simulink model "modeloNoLinealEcuaciones"  (Simulink 7.9)
settings: Solver=ode45  StartTime=0.0  StopTime=300  RelTol=1e-3
values from neighbouring files (symbols this model uses):
  K = lqr(A,B,Q,R)    [LQR.m]    (also in bestQ.m = setK_lqr(Q_i); graficosPenduloReal.m = setK_lqr(Q_optimo))
settings Model: Creator=gdiazh  LastModifiedBy=root
settings OptimizationCC: InitFltsAndDblsToZero=on
settings DebuggingCC: FcnCallInpInsideContextMsg=Use local settings  StrictBusMsg=Warning
settings SFSimCC: SimParseCustomCode=off
settings GRTTargetCC: CombineOutputUpdateFcns=off  GRTInterface=on

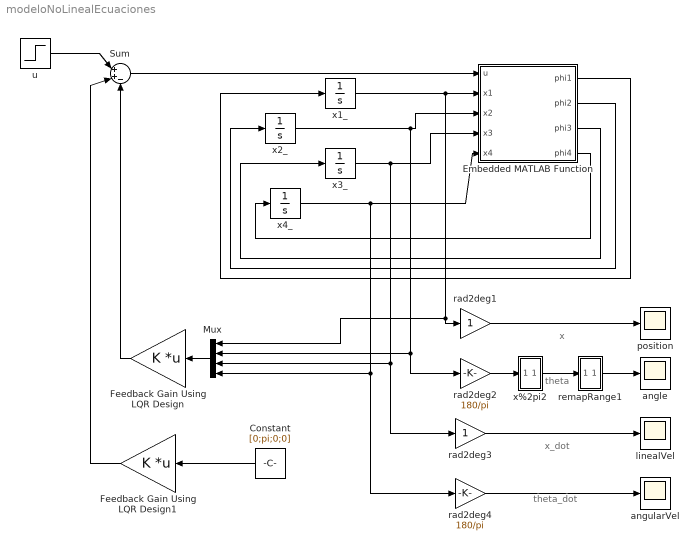
== system modeloNoLinealEcuaciones ==
  note: x
  note: theta
  note: x_dot
  note: theta_dot
  Constant : Constant  Value=[0;pi;0;0]  VectorParams1D=off
  Embedded MATLAB Function : MATLAB Function  TreatAsAtomicUnit=on
  Feedback Gain Using LQR Design : Gain  Gain=K  Multiplication=Matrix(K*u) (u vector)
  Feedback Gain Using LQR Design1 : Gain  Gain=K  Multiplication=Matrix(K*u) (u vector)
  Mux : Mux
  Sum : Sum  Inputs=|++-
  angle : Scope
      settings: TimeRange=0.35  YMin=89.75  YMax=90.25  SaveName=angle
  angularVel : Scope
      settings: SaveName=angularVel
  linealVel : Scope
      settings: SaveName=linealVel
  position : Scope
      settings: SaveName=position
  rad2deg1 : Gain  SaturateOnIntegerOverflow=on  OutDataTypeStr=Inherit: Same as input  ParamDataTypeStr=Inherit: Same as input
  rad2deg2 : Gain  Gain=180/pi  SaturateOnIntegerOverflow=on  OutDataTypeStr=Inherit: Same as input  ParamDataTypeStr=Inherit: Same as input
  rad2deg3 : Gain  SaturateOnIntegerOverflow=on  OutDataTypeStr=Inherit: Same as input  ParamDataTypeStr=Inherit: Same as input
  rad2deg4 : Gain  Gain=180/pi  SaturateOnIntegerOverflow=on  OutDataTypeStr=Inherit: Same as input  ParamDataTypeStr=Inherit: Same as input
  remapRange1 : MATLAB Function  TreatAsAtomicUnit=on
  u : Step  Time=0  After=4.7/1.88  SampleTime=0
  x%2pi2 : MATLAB Function  TreatAsAtomicUnit=on
  x1_ : Integrator  UpperSaturationLimit=50  LowerSaturationLimit=-50
  x2_ : Integrator  InitialCondition=200*pi/180  UpperSaturationLimit=2*pi  LowerSaturationLimit=0
  x3_ : Integrator  UpperSaturationLimit=100  LowerSaturationLimit=-100
  x4_ : Integrator  UpperSaturationLimit=100  LowerSaturationLimit=-100
  wires:
  Sum/1 -> Embedded MATLAB Function/1(u)
  Embedded MATLAB Function/1(phi1) -> x1_/1
  Embedded MATLAB Function/2(phi2) -> x2_/1
  Embedded MATLAB Function/3(phi3) -> x3_/1
  Embedded MATLAB Function/4(phi4) -> x4_/1
  rad2deg4/1 -> angularVel/1
  rad2deg3/1 -> linealVel/1
  rad2deg1/1 -> position/1
  remapRange1/1(y) -> angle/1
  x1_/1 -> Embedded MATLAB Function/2(x1), rad2deg1/1, Mux/1
  x2_/1 -> Embedded MATLAB Function/3(x2), rad2deg2/1, Mux/2
  x3_/1 -> Embedded MATLAB Function/4(x3), rad2deg3/1, Mux/3
  x4_/1 -> Embedded MATLAB Function/5(x4), rad2deg4/1, Mux/4
  rad2deg2/1 -> x%2pi2/1(u)
  x%2pi2/1(y) -> remapRange1/1(value)
  u/1 -> Sum/1
  Mux/1 -> Feedback Gain Using LQR Design/1
  Feedback Gain Using LQR Design/1 -> Sum/3
  Feedback Gain Using LQR Design1/1 -> Sum/2
  Constant/1 -> Feedback Gain Using LQR Design1/1

== matlab function Embedded MATLAB Function ==
  data: u input double; x1 input double; x2 input double; x3 input double; x4 input double; phi1 output double; phi2 output double; phi3 output double; phi4 output double
function [phi1, phi2, phi3, phi4] = fcn(u, x1, x2, x3, x4)
    % This block supports the Embedded MATLAB subset.
    % See the help menu for details. 
    %Valores de los parametros
    g = 9.81;	%[m/s^2]
    M = 0.768;	%[Kg]
    m = 0.104;	%[Kg]
    l = 0.3213;	%[m]
    b = 0.05;	%[Ns/m]
    I = 0.0138;	%[Kg m^2]
    
    phi1 = x3;
    phi2 = x4;
    
    numerador = 1.88*u - 4.7 + m*l*(x4.^(2)).*sin(x2)-(b+0.548).*x3+(M+m)*g*tan(x2);
    denominador = ((M+m)*(I+m*l^2)-(m^2)*(l^2).*(cos(x2).*cos(x2)));
    
    phi3 = (I+m*l^2)*(numerador./denominador)-g*tan(x2);
    phi4 = -(numerador./denominador)*m*l.*cos(x2);
end

== matlab function remapRange1 ==
  data: value input double; y output double
function y = remapRange(value)
    scaleFactor = 1;
    if (value>180*scaleFactor)
        %constants
        fromLow = 181*scaleFactor;
        fromHigh = 360*scaleFactor;
        toLow = -179*scaleFactor;
        toHigh = 0*scaleFactor;
        %calculations
        new_range = toHigh-toLow;
        old_range = fromHigh - fromLow;
        new_value = (new_range/old_range)*(value-fromLow)+toLow;
        y = new_value;
    else
        y = value;
    end
        
end

== matlab function x%2pi2 ==
  data: u input double; y output double
function y = fcn(u)
%#codegen
    y = mod(u,360);
end
